simulink model "FSM_1"  (R2024b)
settings: Solver=VariableStepAuto  StartTime=0.0  StopTime=10.0  RelTol=1e-3
settings Model: Creator=leon-  LastModifiedBy=leon-

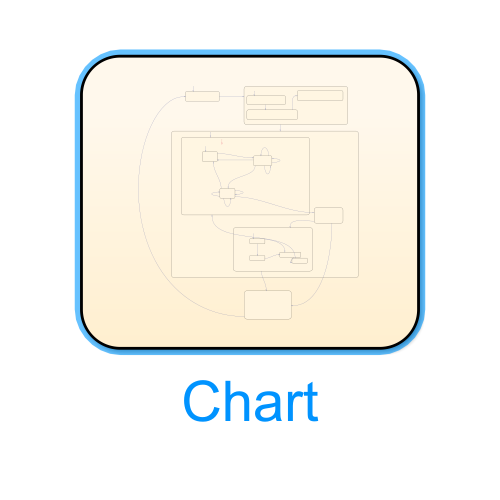
[thumbnail: Simulink's stored preview of the top-level diagram]
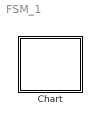
== system FSM_1 ==
  Chart : Stateflow chart  TreatAsAtomicUnit=on

== stateflow chart FSM_1/Chart ==
  state Idle
    display_line1 = "Press any Button";
    display_line2 = "for Reload Pos.";
  state Difficulty_Selection
    state Selected_Difficulty
      display_line1 = 'Selected Diff:';
      display_line2 = ['Level: ' num2str(difficulty_value)];
    state Inital_Difficulty
      display_line1 = "Difficuly";
      display_line2 = "Selection";
    state Change_Difficulty
      display_line1 = "Press Red: Change";
      display_line2 = "Press Blue: Start";
    (default) -> Inital_Difficulty : {timer = 0}
    Change_Difficulty -> Selected_Difficulty : [red_button]{changeLevel()}
    Inital_Difficulty -> Change_Difficulty : [timer > 3]
  state Reloading_Magazine
    state Move_back_to_Mag_Position
      move_to_mag(reload);
    state Move_to_Reloading_Position
      if (~limit_switch1){
      motor(dir = 1, speed = 10);
      }
      if (limit_switch1){
      move_to_reload(mag);
      }
    state Reload
      display_line1 = "Press any Button";
      display_line2 = "when done Reloading";
    (default) -> Move_to_Reloading_Position
    Reload -> Move_back_to_Mag_Position : [red_button || blue_button]
    Move_to_Reloading_Position -> Reload : [limit_switch2]
  state In_Game
    state Human_Turn
      display_line1 = "Waiting for";
      display_line2 = "your Move";
      if (IR ~= IR_triggered){
      IR_triggered = IR;
      timer = 0;
      }
    state Game_Engine
      display_line1 = "Computing";
      display_line2 = "AI Move";
      updateBoard(human_col);
      AI_col = getBestMove();
    state AI_Turn
      display_line1 = "Machine executes";
      display_line2 = "Move";
      state Move_to_Mag
        motor_to_mag(AI_col)
      state Positioning
      state Initial_Move_to_Mag
        motor(dir = -1, speed = 10);
      state Move_to_AI_col
        motor_to_col(AI_col);
      (default) -> Positioning
      Move_to_AI_col -> Move_to_Mag : [complete]{~electromagnet}
      Positioning -> Move_to_AI_col [order 2] : [limit_switch1]{electromagnet}
      Positioning -> Initial_Move_to_Mag [order 1] : [~limit_switch1]
      Initial_Move_to_Mag -> Move_to_AI_col : [limit_switch1]{elecromagnet}
    (default) -> Human_Turn
    Human_Turn -> Game_Engine : [timer > 2]{human_col = IR_triggered}
    Game_Engine -> AI_Turn [order 1] : [complete]
    Move_to_Mag -> Human_Turn : [limit_switch1]
  state Game_Finish
    if (winner == "Draw") {
    display_line1 = "It's a Draw!";
    display_line2 = "";}
    else {
    display_line1 = "The winner is";
    display_line2 = winner;}
  (default) -> Idle
  Game_Finish -> Idle : [red_button || blue_button]
  Idle -> Reloading_Magazine : [red_button || blue_button]
  Move_back_to_Mag_Position -> Difficulty_Selection : [limit_switch1]
  Difficulty_Selection -> In_Game : [blue_button]
  Game_Engine -> Game_Finish [order 2] : [is_winning_move(board, 2)]{winner = "You"}
  AI_Turn -> Game_Finish [order 2] : [is_draw(board)]{winner = "Draw"}
  AI_Turn -> Game_Finish [order 1] : [is_winning_move(board, 1)]{winner = "Machine"}
  data: IR parameter; timer local
